simulink model "SmallPerturbationLinearizedModelHover"  (R2019b)
settings: Solver=ode4  StartTime=0.0  StopTime=100  FixedStep=1e-3
libraries: simulink x1
settings Model: Creator=bitgar  LastModifiedBy=zczhu

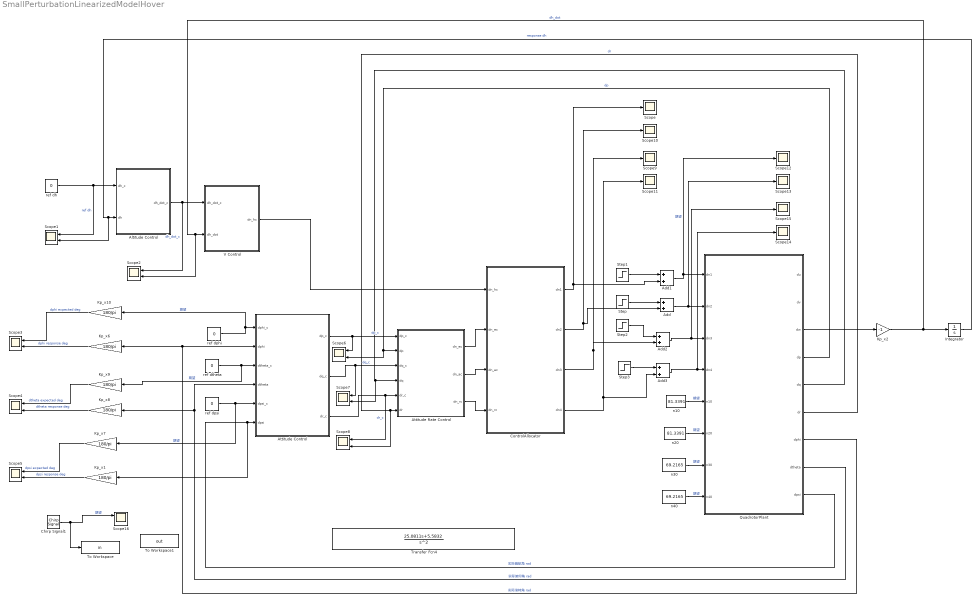
== system SmallPerturbationLinearizedModelHover ==
  Add{,1..3} (4 alike) : Sum
  Altitude Control : Subsystem
  Attitude Control : Subsystem
  Attitude Rate Control : Subsystem
  Chirp Signal1 : simulink/Sources/Chirp Signal  f1=0.001  T=100  f2=5
  ControlAllocator : Subsystem
  Integrator : Integrator
  Kp_x{1,6..10} (6 alike) : Gain  Gain=180/pi
  Kp_x2 : Gain  Gain=-1
  QuadrotorPlant : Subsystem
  Scope{,9..15} (8 alike) : Scope
  Scope{1..8,16} (9 alike) : Scope  NumInputPorts=2
  Step : Step  Time=10  After=0  SampleTime=0
  Step1 : Step  Time=30  After=5  SampleTime=0
  Step2 : Step  Time=10  After=5  SampleTime=0
  Step3 : Step  Time=10  After=5  SampleTime=0
  To Workspace : ToWorkspace  VariableName=in  SampleTime=-1
  To Workspace1 : ToWorkspace  VariableName=out  SampleTime=-1
  Transfer Fcn4 : TransferFcn  Numerator=[0 25.0811 5.5832]  Denominator=[1 0 0]
  V Control : Subsystem
  n10 : Constant  Value=81.3391
  n20 : Constant  Value=81.3391
  n30 : Constant  Value=69.2165
  n40 : Constant  Value=69.2165
  ref dh : Constant  Value=0
  ref dphi : Constant  Value=0
  ref dpsi : Constant  Value=0
  ref dtheta : Constant  Value=0
  wires:
  Chirp Signal1/1 -> Scope16/1, To Workspace/1  "期望"
  Kp_x6/1 -> Scope3/2  "dphi response deg"
  Kp_x8/1 -> Scope4/2  "dtheta response deg"
  ControlAllocator/2(dn2) -> Add/2, Scope10/1
  ControlAllocator/3(dn3) -> Add2/2, Scope9/1
  ControlAllocator/4(dn4) -> Add3/2, Scope11/1
  QuadrotorPlant/4(dp) -> Scope6/2, Attitude Rate Control/2(dp)  "dp"
  QuadrotorPlant/6(dr) -> Scope8/2, Attitude Rate Control/6(dr)  "dr"
  QuadrotorPlant/7(dphi) -> Attitude Control/2(dphi), Kp_x6/1  "实际滚转角 rad"
  QuadrotorPlant/8(dtheta) -> Attitude Control/4(dtheta), Kp_x8/1  "实际俯仰角 rad"
  QuadrotorPlant/9(dpsi) -> Attitude Control/6(dpsi), Kp_x1/1  "实际偏航角 rad"
  ref dphi/1 -> Kp_x10/1, Attitude Control/1(dphi_c)  "期望"
  ref dtheta/1 -> Kp_x9/1, Attitude Control/3(dtheta_c)  "期望"
  n10/1 -> QuadrotorPlant/5(n10)  "期望"
  n20/1 -> QuadrotorPlant/6(n20)  "期望"
  n30/1 -> QuadrotorPlant/7(n30)  "期望"
  Kp_x1/1 -> Scope5/2  "dpsi response deg"
  Kp_x7/1 -> Scope5/1  "dpsi expected deg"
  Kp_x9/1 -> Scope4/1  "dtheta expected deg"
  Kp_x10/1 -> Scope3/1  "dphi expected deg"
  ref dh/1 -> Scope1/1, Altitude Control/1(dh_c)  "ref dh"
  Altitude Control/1(dh_dot_c) -> Scope2/1, V Control/1(dh_dot_c)  "dh_dot_c"
  V Control/1(dn_hc) -> ControlAllocator/1(dn_hc)
  QuadrotorPlant/3(dw) -> Kp_x2/1
  Integrator/1 -> Scope1/2, Altitude Control/2(dh)  "response dh"
  Kp_x2/1 -> Scope2/2, V Control/2(dh_dot), Integrator/1  "dh_dot"
  n40/1 -> QuadrotorPlant/8(n40)  "期望"
  ControlAllocator/1(dn1) -> Add1/2, Scope/1
  Step/1 -> Add/1
  Step1/1 -> Add1/1
  Add1/1 -> Scope12/1, QuadrotorPlant/1(dn1)  "期望"
  Add/1 -> Scope13/1, QuadrotorPlant/2(dn2)
  Step2/1 -> Add2/1
  Step3/1 -> Add3/1
  Add2/1 -> Scope15/1, QuadrotorPlant/3(dn3)
  Add3/1 -> Scope14/1, QuadrotorPlant/4(dn4)
  QuadrotorPlant/5(dq) -> Scope7/2, Attitude Rate Control/4(dq)
  Attitude Rate Control/1(dn_ec) -> ControlAllocator/2(dn_ec)
  Attitude Rate Control/2(dn_ac) -> ControlAllocator/3(dn_ac)
  Attitude Control/2(dq_c) -> Scope7/1, Attitude Rate Control/3(dq_c)  "dq_c"
  Attitude Control/1(dp_c) -> Scope6/1, Attitude Rate Control/1(dp_c)  "dp_c"
  Attitude Rate Control/3(dn_rc) -> ControlAllocator/4(dn_rc)
  Attitude Control/3(dr_c) -> Scope8/1, Attitude Rate Control/5(dr_c)  "dr_c"
  ref dpsi/1 -> Attitude Control/5(dpsi_c), Kp_x7/1  "期望"

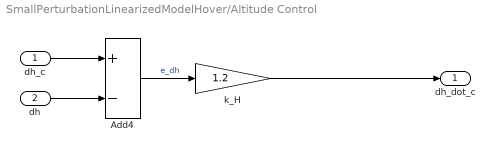
== system SmallPerturbationLinearizedModelHover/Altitude Control ==
  dh_c : Inport
  dh : Inport  Port=2
  Add4 : Sum  Inputs=+-
  k_H : Gain  Gain=1.2
  dh_dot_c : Outport
  wires:
  dh_c/1 -> Add4/1
  dh/1 -> Add4/2
  Add4/1 -> k_H/1  "e_dh"
  k_H/1 -> dh_dot_c/1

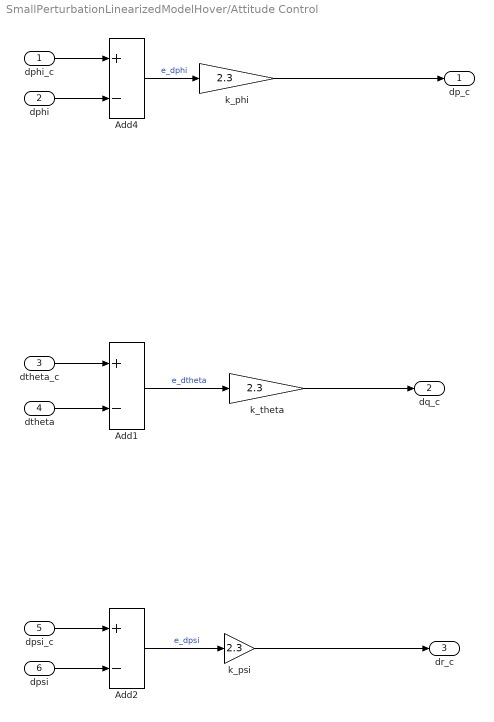
== system SmallPerturbationLinearizedModelHover/Attitude Control ==
  dphi_c : Inport
  dphi : Inport  Port=2
  dtheta_c : Inport  Port=3
  dtheta : Inport  Port=4
  dpsi_c : Inport  Port=5
  dpsi : Inport  Port=6
  Add1 : Sum  Inputs=+-
  Add2 : Sum  Inputs=+-
  Add4 : Sum  Inputs=+-
  k_phi : Gain  Gain=2.3
  k_psi : Gain  Gain=2.3
  k_theta : Gain  Gain=2.3
  dp_c : Outport
  dq_c : Outport  Port=2
  dr_c : Outport  Port=3
  wires:
  dphi_c/1 -> Add4/1
  dphi/1 -> Add4/2
  dtheta_c/1 -> Add1/1
  dtheta/1 -> Add1/2
  dpsi/1 -> Add2/2
  Add4/1 -> k_phi/1  "e_dphi"
  dpsi_c/1 -> Add2/1
  Add1/1 -> k_theta/1  "e_dtheta"
  Add2/1 -> k_psi/1  "e_dpsi"
  k_phi/1 -> dp_c/1
  k_theta/1 -> dq_c/1
  k_psi/1 -> dr_c/1

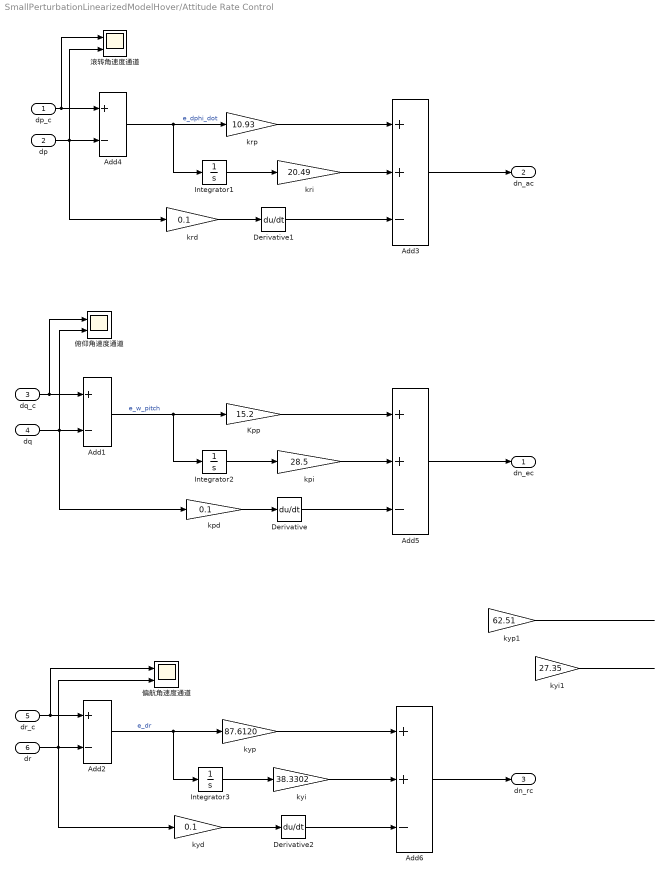
== system SmallPerturbationLinearizedModelHover/Attitude Rate Control ==
  dp_c : Inport
  dp : Inport  Port=2
  dq_c : Inport  Port=3
  dq : Inport  Port=4
  dr_c : Inport  Port=5
  dr : Inport  Port=6
  Add1 : Sum  Inputs=+-
  Add2 : Sum  Inputs=+-
  Add3 : Sum  Inputs=++-
  Add4 : Sum  Inputs=+-
  Add5 : Sum  Inputs=++-
  Add6 : Sum  Inputs=++-
  Derivative : Derivative
  Derivative1 : Derivative
  Derivative2 : Derivative
  Integrator1 : Integrator
  Integrator2 : Integrator
  Integrator3 : Integrator
  Kpp : Gain  Gain=15.2
  kpd : Gain  Gain=0.1
  kpi : Gain  Gain=28.5
  krd : Gain  Gain=0.1
  kri : Gain  Gain=20.49
  krp : Gain  Gain=10.93
  kyd : Gain  Gain=0.1
  kyi : Gain  Gain=38.3302
  kyi1 : Gain  Gain=27.35
  kyp : Gain  Gain=87.6120
  kyp1 : Gain  Gain=62.51
  俯仰角速度通道 : Scope  NumInputPorts=2
  偏航角速度通道 : Scope  NumInputPorts=2
  滚转角速度通道 : Scope  NumInputPorts=2
  dn_ec : Outport
  dn_ac : Outport  Port=2
  dn_rc : Outport  Port=3
  wires:
  dp_c/1 -> 滚转角速度通道/1, Add4/1
  dp/1 -> krd/1, 滚转角速度通道/2, Add4/2
  dq_c/1 -> 俯仰角速度通道/1, Add1/1
  dq/1 -> kpd/1, 俯仰角速度通道/2, Add1/2
  dr/1 -> 偏航角速度通道/2, kyd/1, Add2/2
  Add4/1 -> Integrator1/1, krp/1  "e_dphi_dot"
  dr_c/1 -> 偏航角速度通道/1, Add2/1
  Add3/1 -> dn_ac/1
  kri/1 -> Add3/2
  krp/1 -> Add3/1
  Integrator1/1 -> kri/1
  Integrator2/1 -> kpi/1
  Kpp/1 -> Add5/1
  kpi/1 -> Add5/2
  Add1/1 -> Integrator2/1, Kpp/1  "e_w_pitch"
  Add5/1 -> dn_ec/1
  Add2/1 -> Integrator3/1, kyp/1  "e_dr"
  Integrator3/1 -> kyi/1
  kyp/1 -> Add6/1
  kyi/1 -> Add6/2
  Add6/1 -> dn_rc/1
  kpd/1 -> Derivative/1
  Derivative/1 -> Add5/3
  krd/1 -> Derivative1/1
  Derivative1/1 -> Add3/3
  kyd/1 -> Derivative2/1
  Derivative2/1 -> Add6/3
  ? -> kyi1/1
  kyp1/1 -> ?
  kyi1/1 -> ?

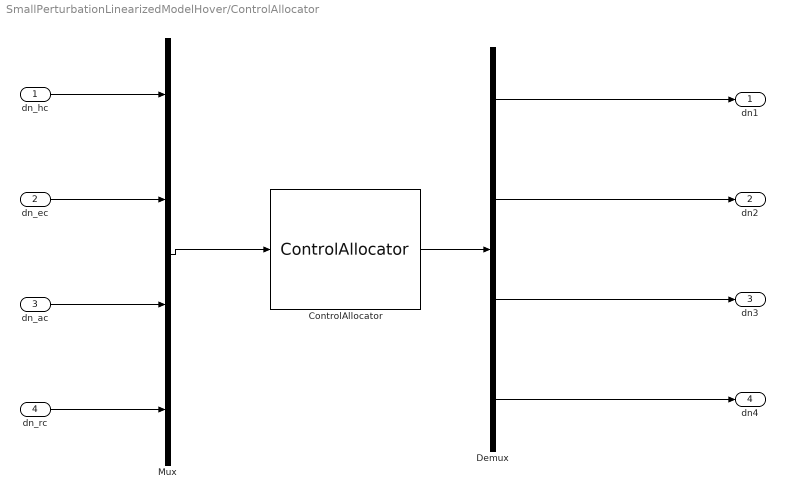
== system SmallPerturbationLinearizedModelHover/ControlAllocator ==
  dn_hc : Inport
  dn_ec : Inport  Port=2
  dn_ac : Inport  Port=3
  dn_rc : Inport  Port=4
  ControlAllocator : S-Function  FunctionName=ControlAllocator  Parameters=0.52 0.7107  SFunctionDeploymentMode=off  EnableBusSupport=off
  Demux : Demux
  Mux : Mux
  dn1 : Outport
  dn2 : Outport  Port=2
  dn3 : Outport  Port=3
  dn4 : Outport  Port=4
  wires:
  Demux/2 -> dn2/1
  Demux/1 -> dn1/1
  Demux/3 -> dn3/1
  Demux/4 -> dn4/1
  Mux/1 -> ControlAllocator/1
  dn_ec/1 -> Mux/2
  dn_ac/1 -> Mux/3
  dn_rc/1 -> Mux/4
  ControlAllocator/1 -> Demux/1
  dn_hc/1 -> Mux/1

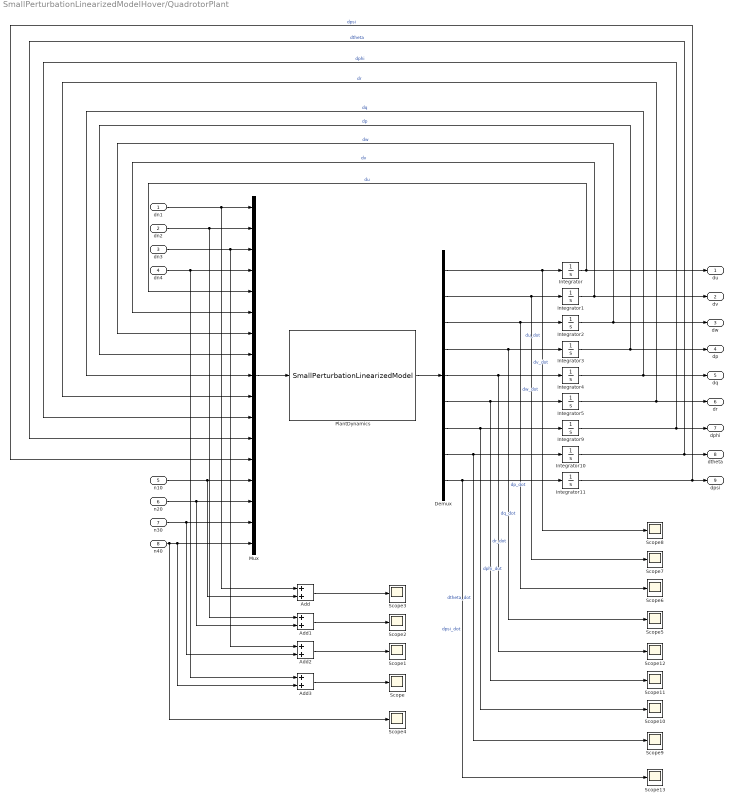
== system SmallPerturbationLinearizedModelHover/QuadrotorPlant ==
  dn1 : Inport
  dn2 : Inport  Port=2
  dn3 : Inport  Port=3
  dn4 : Inport  Port=4
  n10 : Inport  Port=5
  n20 : Inport  Port=6
  n30 : Inport  Port=7
  n40 : Inport  Port=8
  Add{,1..3} (4 alike) : Sum
  Demux : Demux  Outputs=9
  Integrator{,1..5,9..11} (9 alike) : Integrator
  Mux : Mux  Inputs=17
  PlantDynamics : S-Function  FunctionName=SmallPerturbationLinearizedModel  Parameters=40.37 9.81 0.52 0.7107 1.375 1.126 0.0184 8.1701e-04 13.59 9.052 21.238 0.348  SFunctionDeploymentMode=off  EnableBusSupport=off
  Scope{,1..13} (14 alike) : Scope
  du : Outport
  dv : Outport  Port=2
  dw : Outport  Port=3
  dp : Outport  Port=4
  dq : Outport  Port=5
  dr : Outport  Port=6
  dphi : Outport  Port=7
  dtheta : Outport  Port=8
  dpsi : Outport  Port=9
  wires:
  Demux/4 -> Scope5/1, Integrator3/1  "dp_dot"
  Mux/1 -> PlantDynamics/1
  Demux/3 -> Scope6/1, Integrator2/1  "dw_dot"
  dn2/1 -> Add1/1, Mux/2
  Demux/1 -> Scope8/1, Integrator/1  "du_dot"
  Demux/5 -> Scope12/1, Integrator4/1  "dq_dot"
  Demux/6 -> Scope11/1, Integrator5/1  "dr_dot"
  Demux/2 -> Scope7/1, Integrator1/1  "dv_dot"
  dn4/1 -> Add3/1, Mux/4
  dn1/1 -> Add/1, Mux/1
  dn3/1 -> Add2/1, Mux/3
  PlantDynamics/1 -> Demux/1
  Integrator9/1 -> Mux/11, dphi/1  "dphi"
  Integrator10/1 -> Mux/12, dtheta/1  "dtheta"
  Integrator11/1 -> Mux/13, dpsi/1  "dpsi"
  Integrator/1 -> du/1, Mux/5  "du"
  Integrator1/1 -> Mux/6, dv/1  "dv"
  Integrator2/1 -> Mux/7, dw/1  "dw"
  Demux/7 -> Scope10/1, Integrator9/1  "dphi_dot"
  Demux/8 -> Scope9/1, Integrator10/1  "dtheta_dot"
  Demux/9 -> Scope13/1, Integrator11/1  "dpsi_dot"
  Integrator3/1 -> Mux/8, dp/1  "dp"
  Integrator4/1 -> Mux/9, dq/1  "dq"
  Integrator5/1 -> Mux/10, dr/1  "dr"
  n30/1 -> Add2/2, Mux/16
  n10/1 -> Add/2, Mux/14
  n20/1 -> Add1/2, Mux/15
  n40/1 -> Scope4/1, Add3/2, Mux/17
  Add3/1 -> Scope/1
  Add/1 -> Scope3/1
  Add1/1 -> Scope2/1
  Add2/1 -> Scope1/1

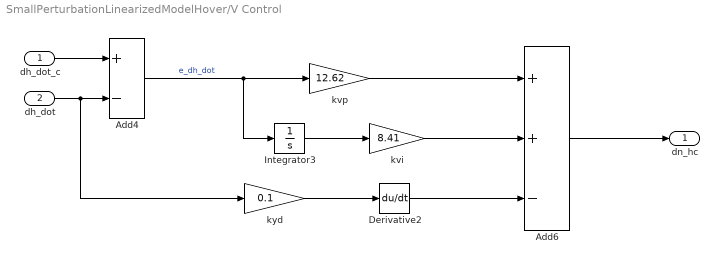
== system SmallPerturbationLinearizedModelHover/V Control ==
  dh_dot_c : Inport
  dh_dot : Inport  Port=2
  Add4 : Sum  Inputs=+-
  Add6 : Sum  Inputs=++-
  Derivative2 : Derivative
  Integrator3 : Integrator
  kvi : Gain  Gain=8.41
  kvp : Gain  Gain=12.62
  kyd : Gain  Gain=0.1
  dn_hc : Outport
  wires:
  dh_dot_c/1 -> Add4/1
  dh_dot/1 -> kyd/1, Add4/2
  Add4/1 -> Integrator3/1, kvp/1  "e_dh_dot"
  Derivative2/1 -> Add6/3
  kyd/1 -> Derivative2/1
  Add6/1 -> dn_hc/1
  kvi/1 -> Add6/2
  Integrator3/1 -> kvi/1
  kvp/1 -> Add6/1
